simulink model "operationalSpacePDControl_compliance"  (R2021a)
settings: Solver=VariableStepAuto  StartTime=0.0  StopTime=5  RelTol=1e-3
values from neighbouring files (symbols this model uses):
  K = diag([0 10 0 0 0 10])    [assignment11_main.m]
  Kd = diag([1, 5, 10, 1, 1, 1])    [assignment11_main.m]
  Kp = diag([10, 20, 20, 50, 50, 50])    [assignment11_main.m]
  x_d = goalPose_0    [assignment11_main.m]
libraries: vrlib x1
settings Model: Creator=fabio  LastModifiedBy=fabio
settings DebuggingCC: UnconnectedInputMsg=none  UnconnectedOutputMsg=none

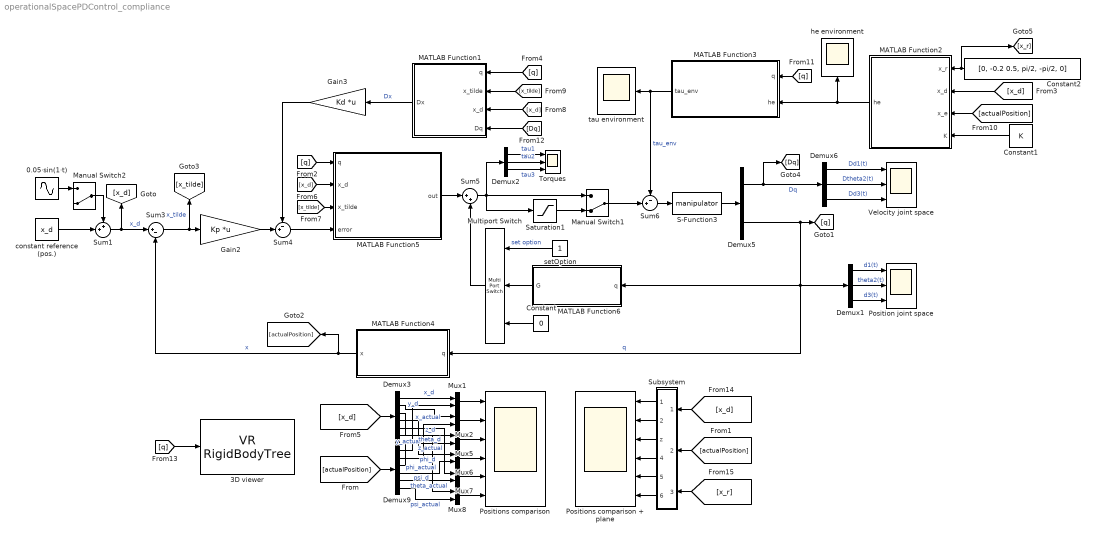
== system operationalSpacePDControl_compliance ==
  "0.05·sin(1·t) " : Sin  Amplitude=0.05  SampleTime=0
  3D viewer : vrlib/VR RigidBodyTree  RBT=robot  useRBT=off  Ts=0.5  ForceViewerOpen=on
      settings: SourceProductBaseCode=SL
  Constant : Constant  Value=0
  Constant1 : Constant  Value=K  VectorParams1D=off
  Constant2 : Constant  Value=[0, -0.2 0.5, pi/2, -pi/2, 0]
  Demux1 : Demux  Outputs=3
  Demux2 : Demux  Outputs=3
  Demux3 : Demux  Outputs=6
  Demux5 : Demux  Outputs=2
  Demux6 : Demux  Outputs=3
  Demux9 : Demux  Outputs=6
  Gain2 : Gain  Gain=Kp  Multiplication=Matrix(K*u) (u vector)
  Gain3 : Gain  Gain=Kd  Multiplication=Matrix(K*u) (u vector)
  MATLAB Function1 : MATLAB Function  TreatAsAtomicUnit=on
  MATLAB Function2 : MATLAB Function  TreatAsAtomicUnit=on
  MATLAB Function3 : MATLAB Function  TreatAsAtomicUnit=on
  MATLAB Function4 : MATLAB Function  TreatAsAtomicUnit=on
  MATLAB Function5 : MATLAB Function  TreatAsAtomicUnit=on
  MATLAB Function6 : MATLAB Function  TreatAsAtomicUnit=on
  Manual Switch1 : ManualSwitch  CurrentSetting=0
  Manual Switch2 : ManualSwitch  CurrentSetting=0
  Multiport Switch : MultiPortSwitch  Inputs=2
  Mux{1..2,5..8} (6 alike) : Mux  Inputs=2
  Position joint space : Scope  NumInputPorts=3
  Positions comparison : Scope  NumInputPorts=6
  Positions comparison + plane : Scope  NumInputPorts=6
  S-Function3 : S-Function  FunctionName=manipulator  Parameters=myRobot  SFunctionDeploymentMode=off  EnableBusSupport=off
  Saturation1 : Saturate  UpperLimit=10  LowerLimit=-10
  Subsystem : Subsystem
  Sum1 : Sum  Inputs=++|
  Sum3 : Sum  Inputs=|+-
  Sum4 : Sum  Inputs=-+|
  Sum5 : Sum  Inputs=|++
  Sum6 : Sum  Inputs=-+|
  Torques : Scope  NumInputPorts=3
  Velocity joint space : Scope  NumInputPorts=3
  constant reference (pos.) : Constant  Value=x_d
  he environment : Scope
  setOption : Constant
  tau environment : Scope
  wires:
  Sum5/1 -> Saturation1/1, Demux2/1, Manual Switch1/1
  Demux9/3 -> Mux5/2  "z_actual"
  Sum3/1 -> Gain2/1, [x_tilde]  "x_tilde"
  Sum1/1 -> Sum3/1, [x_d]  "x_d"
  Demux6/3 -> Velocity joint space/3  "Dd3(t)"
  Demux6/2 -> Velocity joint space/2  "Dtheta2(t)"
  Demux6/1 -> Velocity joint space/1  "Dd1(t)"
  S-Function3/1 -> Demux5/1
  Gain3/1 -> Sum4/1
  Gain2/1 -> Sum4/2
  Multiport Switch/1 -> Sum5/2
  MATLAB Function6/1(G) -> Multiport Switch/2
  Constant/1 -> Multiport Switch/3
  setOption/1 -> Multiport Switch/1  "set option"
  constant reference (pos.)/1 -> Sum1/2
  Demux2/1 -> Torques/1  "tau1"
  Demux2/2 -> Torques/2  "tau2"
  Demux2/3 -> Torques/3  "tau3"
  "0.05·sin(1·t) "/1 -> Manual Switch2/1
  Manual Switch2/1 -> Sum1/1
  [actualPosition] -> Demux9/1
  MATLAB Function5/1(out) -> Sum5/1
  MATLAB Function4/1(x) -> [actualPosition], Sum3/2  "x"
  [x_d] -> Demux3/1
  Demux3/3 -> Mux5/1  "z_d"
  Saturation1/1 -> Manual Switch1/2
  Demux1/1 -> Position joint space/1  "d1(t)"
  Demux1/2 -> Position joint space/2  "theta2(t)"
  Demux1/3 -> Position joint space/3  "d3(t)"
  Demux3/1 -> Mux1/1  "x_d"
  Demux9/1 -> Mux1/2  "x_actual"
  Demux3/2 -> Mux2/1  "y_d"
  Demux9/2 -> Mux2/2  "y_actual"
  Demux3/4 -> Mux6/1  "phi_d"
  Demux9/4 -> Mux6/2  "phi_actual"
  Demux9/5 -> Mux7/2  "theta_actual"
  Demux3/5 -> Mux7/1  "theta_d"
  Demux3/6 -> Mux8/1  "psi_d"
  Demux9/6 -> Mux8/2  "psi_actual"
  Mux1/1 -> Positions comparison/1
  Mux2/1 -> Positions comparison/2
  Mux5/1 -> Positions comparison/3
  Mux6/1 -> Positions comparison/4
  Mux7/1 -> Positions comparison/5
  Mux8/1 -> Positions comparison/6
  MATLAB Function1/1(Dx) -> Gain3/1  "Dx"
  Demux5/1 -> Demux6/1, [Dq]  "Dq"
  [x_d] -> MATLAB Function1/3(x_d)
  [q] -> MATLAB Function1/1(q)
  [x_tilde] -> MATLAB Function1/2(x_tilde)
  [q] -> MATLAB Function5/1(q)
  [x_d] -> MATLAB Function5/2(x_d)
  [x_tilde] -> MATLAB Function5/3(x_tilde)
  Sum4/1 -> MATLAB Function5/4(error)
  Constant2/1 -> [x_r], MATLAB Function2/1(x_r)
  [x_d] -> MATLAB Function2/2(x_d)
  [actualPosition] -> MATLAB Function2/3(x_e)
  Constant1/1 -> MATLAB Function2/4(K)
  MATLAB Function2/1(he) -> MATLAB Function3/2(he), he environment/1
  [q] -> MATLAB Function3/1(q)
  Manual Switch1/1 -> Sum6/2
  Sum6/1 -> S-Function3/1
  MATLAB Function3/1(tau_env) -> tau environment/1, Sum6/1  "tau_env"
  [Dq] -> MATLAB Function1/4(Dq)
  [q] -> 3D viewer/1
  Demux5/2 -> MATLAB Function4/1(q), MATLAB Function6/1(q), Demux1/1, [q]  "q"
  [x_d] -> Subsystem/1(x_d)
  [actualPosition] -> Subsystem/2(x_e)
  [x_r] -> Subsystem/3(x_r)
  Subsystem/1(x) -> Positions comparison + plane/1
  Subsystem/2(y) -> Positions comparison + plane/2
  Subsystem/3(z) -> Positions comparison + plane/3
  Subsystem/4(phi) -> Positions comparison + plane/4
  Subsystem/5(theta) -> Positions comparison + plane/5
  Subsystem/6(psi) -> Positions comparison + plane/6

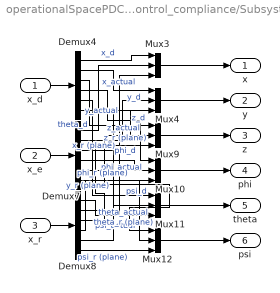
== system operationalSpacePDControl_compliance/Subsystem ==
  x_d : Inport
  x_e : Inport  Port=2
  x_r : Inport  Port=3
  Demux4 : Demux  Outputs=6
  Demux7 : Demux  Outputs=6
  Demux8 : Demux  Outputs=6
  Mux{3..4,9..12} (6 alike) : Mux  Inputs=3
  x : Outport
  y : Outport  Port=2
  z : Outport  Port=3
  phi : Outport  Port=4
  theta : Outport  Port=5
  psi : Outport  Port=6
  wires:
  Demux8/1 -> Mux3/3  "x_r (plane)"
  Demux7/3 -> Mux9/2  "z_actual"
  Demux4/4 -> Mux10/1  "phi_d"
  Demux8/2 -> Mux4/3  "y_r (plane)"
  Demux7/6 -> Mux12/2  "psi_actual"
  Demux7/4 -> Mux10/2  "phi_actual"
  Demux7/1 -> Mux3/2  "x_actual"
  Demux8/3 -> Mux9/3  "z_r (plane)"
  Demux4/3 -> Mux9/1  "z_d"
  Demux4/6 -> Mux12/1  "psi_d"
  Demux4/5 -> Mux11/1  "theta_d"
  Demux7/5 -> Mux11/2  "theta_actual"
  Demux4/2 -> Mux4/1  "y_d"
  Demux4/1 -> Mux3/1  "x_d"
  Demux7/2 -> Mux4/2  "y_actual"
  Demux8/6 -> Mux12/3  "psi_r (plane)"
  Demux8/4 -> Mux10/3  "phi_r (plane)"
  Mux11/1 -> theta/1
  Demux8/5 -> Mux11/3  "theta_r (plane)"
  x_d/1 -> Demux4/1
  x_e/1 -> Demux7/1
  Mux9/1 -> z/1
  Mux12/1 -> psi/1
  Mux10/1 -> phi/1
  Mux4/1 -> y/1
  Mux3/1 -> x/1
  x_r/1 -> Demux8/1

== matlab function operationalSpacePDControl_compliance/MATLAB Function1 ==
  data: q input size=3; x_tilde input; x_d input; Dx output; Dq input size=3
function Dx = Jad_x_Dq(q, x_tilde, x_d, Dq)
    if max(size(q)) < 3
        q = [0 0 0];   
    end  
    if max(size(Dq)) < 3
        Dq = [0 0 0];   
    end  
    J_Ad = get_Jad_matrix(q, x_tilde);                
   
    Dx = J_Ad * Dq;
      
end

== matlab function operationalSpacePDControl_compliance/MATLAB Function2 ==
  data: x_r input; x_d input; x_e input; K input; he output
function he = environment(x_r, x_d, x_e, K)
    
    y_plane = x_r(2); %negative value: -0.2
    
    %contact with the plane
    if max(size(x_e)) > 1 && x_e(2) < y_plane 
        dx_re = x_e - x_r;
        he = K * dx_re;
    else %no contact with the plane
        he = [0 0 0 0 0 0].';
    end
end

== matlab function operationalSpacePDControl_compliance/MATLAB Function3 ==
  data: q input; he input; tau_env output
function tau_env = Jg_transposed(q, he)
    if max(size(q)) < 3
        q = [0 0 0];   
    end  
    
    %Geometric jacobian w.r.t. to frame 0
    Jg = get_Jg_matrix(q);
                   
    tau_env = Jg.' * he;           
      
end

== matlab function operationalSpacePDControl_compliance/MATLAB Function4 ==
  data: q input; x output
function x = k(q) 
    %Compute the direct kinematics from last transformation matrix
    if max(size(q)) < 3
        q = [0 0 0];   
    end
    
    %get rotation matrix and translation vector from ∑0 to ∑ee   
    T0_to_ee = get_T0_ee_matrix(q);
    R0_to_ee = T0_to_ee(1:3,1:3);
    p0_to_ee = T0_to_ee(1:3,4);    
                 
    eulerAngles = rotm2eul(R0_to_ee, 'ZYZ');
  
    x = [ p0_to_ee;
          eulerAngles.' ]; %return complete direct kinematics
    
end

== matlab function operationalSpacePDControl_compliance/MATLAB Function5 ==
  data: q input; x_d input; out output; x_tilde input; error input
function out = Jad_transposed(q, x_d, x_tilde, error)
    if max(size(q)) < 3
        q = [0 0 0];   
    end  

    J_Ad = get_Jad_matrix(q, x_tilde);      
                 
    out = J_Ad.' * error;
                 
      
end

== matlab function operationalSpacePDControl_compliance/MATLAB Function6 ==
  data: q input; G output
function G = gravityTerm(q) 
    if max(size(q)) < 3
        q = [0 0 0];   
    end 
    G = get_G_matrix(q);
end
